simulink model "modelo_ventilador_difuso"  (R2025a)
settings: Solver=VariableStepAuto  StartTime=0.0  StopTime=500  RelTol=1e-3
values from neighbouring files (symbols this model uses):
  alpha_H = 0.06    [parametros_ventilador.m]
  alpha_T = 0.08    [parametros_ventilador.m]
  beta_H = 0.03    [parametros_ventilador.m]
  beta_T = 0.02    [parametros_ventilador.m]
  H0 = 70    [parametros_ventilador.m]
  H_ext = 45    [parametros_ventilador.m]
  H_ref = 50    [parametros_ventilador.m]
  Q_int = 2    [parametros_ventilador.m]
  T0 = 30    [parametros_ventilador.m]
  T_ext = 22    [parametros_ventilador.m]
  T_ref = 24    [parametros_ventilador.m]
  tau_H = 40    [parametros_ventilador.m]
  tau_T = 30    [parametros_ventilador.m]
  Ts = 1    [parametros_ventilador.m]
  W_int = 1    [parametros_ventilador.m]
libraries: fuzblock x1
settings Model: Creator=sonic  LastModifiedBy=sonic

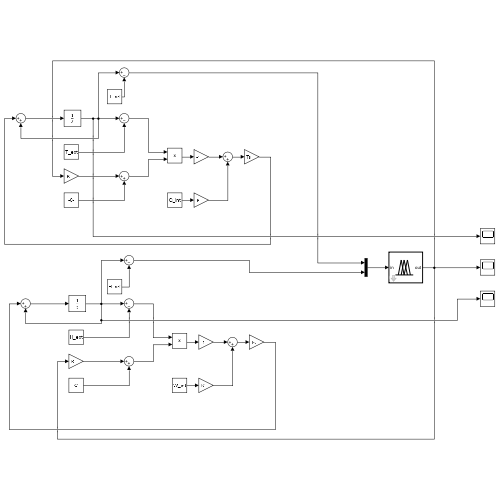
[thumbnail: Simulink's stored preview of the top-level diagram]
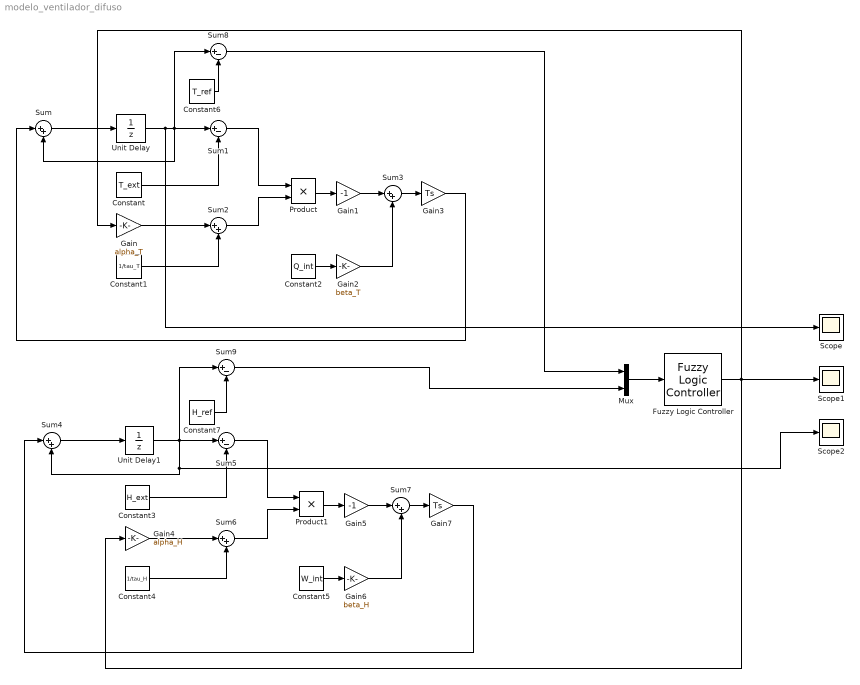
== system modelo_ventilador_difuso ==
  Constant : Constant  Value=T_ext
  Constant1 : Constant  Value=1/tau_T
  Constant2 : Constant  Value=Q_int
  Constant3 : Constant  Value=H_ext
  Constant4 : Constant  Value=1/tau_H
  Constant5 : Constant  Value=W_int
  Constant6 : Constant  Value=T_ref
  Constant7 : Constant  Value=H_ref
  Fuzzy Logic Controller : fuzblock/Fuzzy Logic  Controller  FIS='control_ventilador.fis'  OutputSampleNumber=101  DataType=double  UseLookupTable=off  NumBreakpoints=10  FuzzifiedInputs=off  RuleFiringStrengths=off  RuleOutputs=off  AggregatedOutputs=off  SimulateUsing=Interpreted execution  OutOfRangeInputValueMessage=warning  NoRuleFiredMessage=warning  EmptyOutputFuzzySetMessage=warning
  Gain : Gain  Gain=alpha_T
  Gain1 : Gain  Gain=-1
  Gain2 : Gain  Gain=beta_T
  Gain3 : Gain  Gain=Ts
  Gain4 : Gain  Gain=alpha_H
  Gain5 : Gain  Gain=-1
  Gain6 : Gain  Gain=beta_H
  Gain7 : Gain  Gain=Ts
  Mux : Mux  Inputs=2
  Product : Product
  Product1 : Product
  Scope : Scope
      settings: ActiveDisplayYMinimum=22.011929005298146  ActiveDisplayYMaximum=30.887563443855761
  Scope1 : Scope
      settings: ActiveDisplayYMinimum=0.079298557420698856  ActiveDisplayYMaximum=0.64530977982830984
  Scope2 : Scope
      settings: ActiveDisplayYMinimum=42.886929919928761  ActiveDisplayYMaximum=73.012563342230138  DataLoggingVariableName=ScopeData2
  Sum{,2..4,6..7} (6 alike) : Sum  Inputs=|++
  Sum{1,5,8..9} (4 alike) : Sum  Inputs=|+-
  Unit Delay : UnitDelay  InitialCondition=T0  SampleTime=Ts  HasFrameUpgradeWarning=on
  Unit Delay1 : UnitDelay  InitialCondition=H0  SampleTime=Ts  HasFrameUpgradeWarning=on
  wires:
  Sum/1 -> Unit Delay/1
  Unit Delay/1 -> Scope/1, Sum/2, Sum1/1, Sum8/1
  Constant/1 -> Sum1/2
  Constant1/1 -> Sum2/2
  Gain/1 -> Sum2/1
  Sum1/1 -> Product/1
  Sum2/1 -> Product/2
  Product/1 -> Gain1/1
  Constant2/1 -> Gain2/1
  Gain1/1 -> Sum3/1
  Gain2/1 -> Sum3/2
  Sum3/1 -> Gain3/1
  Gain3/1 -> Sum/1
  Gain7/1 -> Sum4/1
  Gain6/1 -> Sum7/2
  Gain5/1 -> Sum7/1
  Product1/1 -> Gain5/1
  Constant4/1 -> Sum6/2
  Sum6/1 -> Product1/2
  Unit Delay1/1 -> Scope2/1, Sum4/2, Sum9/1, Sum5/1
  Sum4/1 -> Unit Delay1/1
  Sum7/1 -> Gain7/1
  Constant3/1 -> Sum5/2
  Sum5/1 -> Product1/1
  Constant5/1 -> Gain6/1
  Gain4/1 -> Sum6/1
  Constant6/1 -> Sum8/2
  Constant7/1 -> Sum9/2
  Sum9/1 -> Mux/2
  Sum8/1 -> Mux/1
  Mux/1 -> Fuzzy Logic Controller/1
  Fuzzy Logic Controller/1 -> Scope1/1, Gain4/1, Gain/1
